simulink model "FlightCore"  (R2025b)
settings: Solver=FixedStepDiscrete  StartTime=0.0  StopTime=10  FixedStep=0.001  RelTol=1e-3
libraries: simulink x1
settings Model: DataDictionary=GlobalTypes.sldd  Creator=89447  LastModifiedBy=89447
settings OptimizationCC: DefaultParameterBehavior=Inlined  EnhancedBackFolding=on  PassReuseOutputArgsAs=Individual arguments  ZeroExternalMemoryAtStartup=off  ZeroInternalMemoryAtStartup=off  MaxStackSize=64  OptimizeBlockOrder=speed  DifferentSizesBufferReuse=on  OptimizationCustomize=off  EfficientTunableParamExpr=on
settings HardwareCC: ProdBitPerLong=64.0  ProdHWDeviceType=Intel->x86-64 (Linux 64)
settings SFSimCC: MATLABDynamicMemAlloc=off
settings RTWCC: SystemTargetFile=ert.tlc  HardwareBoard=Robot Operating System 2 (ROS 2)  TLCOptions="-aInlineSetEventsForThisBaseRateFcn=TLC_FALSE -aSuppressMultiTaskScheduler=TLC_FALSE  -aRateBasedStepFcn=0"  TemplateMakefile=ert_default_tmf  Toolchain=Colcon Tools  TargetLang=C++  Description=Embedded Coder
settings CodeAppCC: ForceParamTrailComments=on  IgnoreCustomStorageClasses=off  OperatorAnnotations=on  SimulinkDataObjDesc=on  SFDataObjDesc=on  InsertBlockDesc=on
settings ERTTargetCC: ExtModeTransport=2.0  ExtModeStaticAlloc=on  ExtModeMexFile=ext_xcp  ExtModeIntrfLevel=Level2 - Open  RootIOFormat=Structure reference  TargetLangStandard=C++11 (ISO)  SupportContinuousTime=on

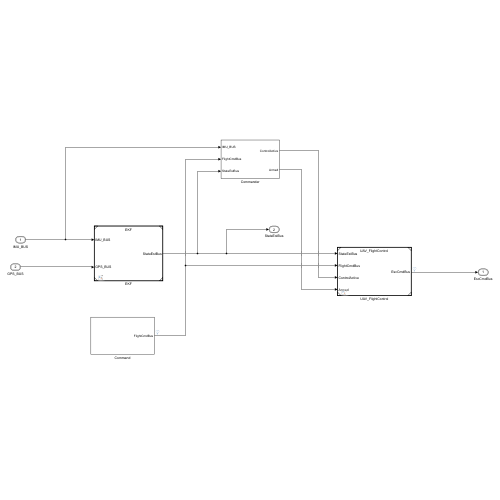
[thumbnail: Simulink's stored preview of the top-level diagram]
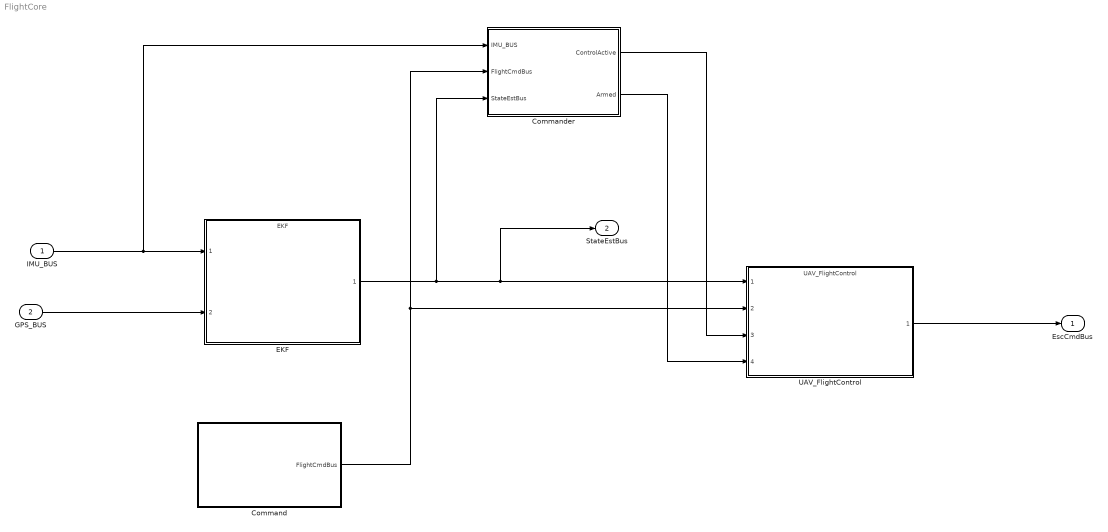
== system FlightCore ==
  IMU_BUS : Inport  OutDataTypeStr=Bus: IMU_BUS
  GPS_BUS : Inport  Port=2  OutDataTypeStr=Bus: GPS_BUS
  Command : Subsystem
  Commander : Subsystem
  EKF : ModelReference  ModelNameDialog=EKF  SimulationMode=Normal  ModelReferenceVersion=4.30
  UAV_FlightControl : ModelReference  ModelNameDialog=UAV_FlightControl  SimulationMode=Normal  ModelReferenceVersion=4.42
  EscCmdBus : Outport  OutDataTypeStr=Bus: EscCmdBus
  StateEstBus : Outport  Port=2  OutDataTypeStr=Bus: StateEstBus
  wires:
  GPS_BUS/1 -> EKF/2
  IMU_BUS/1 -> Commander/1(IMU_BUS), EKF/1
  UAV_FlightControl/1 -> EscCmdBus/1
  EKF/1 -> Commander/3(StateEstBus), UAV_FlightControl/1, StateEstBus/1
  Command/1(FlightCmdBus) -> UAV_FlightControl/2, Commander/2(FlightCmdBus)
  Commander/1(ControlActive) -> UAV_FlightControl/3
  Commander/2(Armed) -> UAV_FlightControl/4

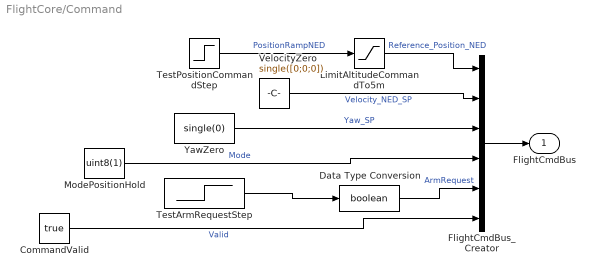
== system FlightCore/Command ==
  CommandValid : Constant  Value=true  OutDataTypeStr=boolean  SampleTime=0.001
  Data Type Conversion : DataTypeConversion  OutDataTypeStr=boolean  SaturateOnIntegerOverflow=off  RndMeth=Floor
  FlightCmdBus_Creator : BusCreator  Inputs=6  OutDataTypeStr=Bus: FlightCmdBus  NonVirtualBus=on
      settings: InheritFromInputs=off
  LimitAltitudeCommandTo5m : Saturate  UpperLimit=single([0;0;0])  LowerLimit=single([0;0;-5])  OutDataTypeStr=single
  ModePositionHold : Constant  Value=uint8(1)  SampleTime=0.001
  TestArmRequestStep : Step  OutDataTypeStr=single  SampleTime=0.001
  TestPositionCommandStep : Step  Time=5  Before=single([0;0;0])  After=single([0;0;-5])  SampleTime=0
  VelocityZero : Constant  Value=single([0;0;0])
  YawZero : Constant  Value=single(0)  SampleTime=0.001
  FlightCmdBus : Outport  OutDataTypeStr=Bus: FlightCmdBus  BusOutputAsStruct=on
  wires:
  FlightCmdBus_Creator/1 -> FlightCmdBus/1
  CommandValid/1 -> FlightCmdBus_Creator/6  "Valid"
  ModePositionHold/1 -> FlightCmdBus_Creator/4  "Mode"
  YawZero/1 -> FlightCmdBus_Creator/3  "Yaw_SP"
  TestArmRequestStep/1 -> Data Type Conversion/1
  Data Type Conversion/1 -> FlightCmdBus_Creator/5  "ArmRequest"
  LimitAltitudeCommandTo5m/1 -> FlightCmdBus_Creator/1  "Reference_Position_NED"
  TestPositionCommandStep/1 -> LimitAltitudeCommandTo5m/1  "PositionRampNED"
  VelocityZero/1 -> FlightCmdBus_Creator/2  "Velocity_NED_SP"

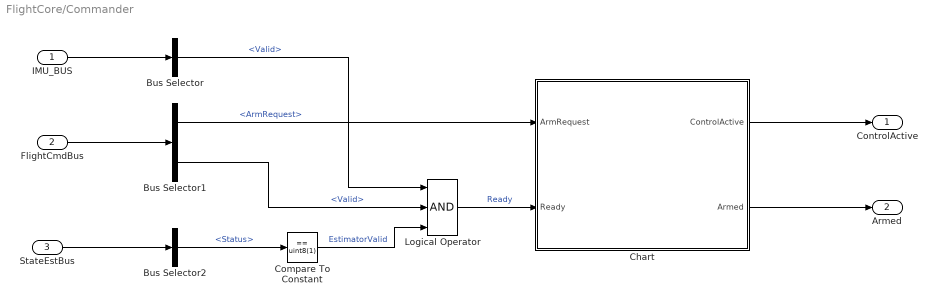
== system FlightCore/Commander ==
  IMU_BUS : Inport  OutDataTypeStr=Bus: IMU_BUS
  FlightCmdBus : Inport  Port=2  OutDataTypeStr=Bus: FlightCmdBus
  StateEstBus : Inport  Port=3  OutDataTypeStr=Bus: StateEstBus
  Bus Selector : BusSelector  OutputSignals=Valid
  Bus Selector1 : BusSelector  OutputSignals=ArmRequest,Valid
  Bus Selector2 : BusSelector  OutputSignals=Status
  Chart : Stateflow chart  TreatAsAtomicUnit=on
  Compare To Constant : simulink/Logic and Bit Operations/Compare To Constant  relop===  const=uint8(1)  OutDataTypeStr=boolean
  Logical Operator : Logic  Inputs=3  AllPortsSameDT=off  OutDataTypeStr=boolean
  ControlActive : Outport
  Armed : Outport  Port=2
  wires:
  StateEstBus/1 -> Bus Selector2/1
  FlightCmdBus/1 -> Bus Selector1/1
  IMU_BUS/1 -> Bus Selector/1
  Bus Selector/1 -> Logical Operator/1  "<Valid>"
  Bus Selector1/2 -> Logical Operator/2  "<Valid>"
  Bus Selector2/1 -> Compare To Constant/1  "<Status>"
  Bus Selector1/1 -> Chart/1(ArmRequest)  "<ArmRequest>"
  Compare To Constant/1 -> Logical Operator/3  "EstimatorValid"
  Logical Operator/1 -> Chart/2(Ready)  "Ready"
  Chart/2(Armed) -> Armed/1
  Chart/1(ControlActive) -> ControlActive/1

== stateflow chart FlightCore/Commander/Chart ==
  state DISARMED
    entry:
    Armed = false;
    ControlActive = false;
    during:
    Armed = false;
    ControlActive = false;
  state ACTIVE
    entry:
    Armed = true;
    ControlActive = true;
    during:
    Armed = true;
    ControlActive = true;
  state CONTROL_INHIBITED
    entry:
    Armed = true;
    ControlActive = false;
    during:
    Armed = true;
    ControlActive = false;
  (default) -> DISARMED
  DISARMED -> ACTIVE : [rising(ArmRequest) && Ready]
  ACTIVE -> DISARMED [order 1] : [~ArmRequest]
  CONTROL_INHIBITED -> DISARMED : [~ArmRequest]
  ACTIVE -> CONTROL_INHIBITED [order 2] : [ArmRequest && ~Ready]
  data: ControlActive output; ArmRequest input; Ready input; Armed output
